simulink model "flightControlSystem"  (R2022b)
settings: Solver=ode3  StartTime=0  StopTime=TFinal  FixedStep=Ts  RelTol=1e-3  EnableMultiTasking=on
undefined symbols (not defined in the file): codertarget, Controller, DiscIntNeverNeededParam, Discrete, Estimator, g, init, Sensors, Time, Ts, var_acc_angle_N, var_bias_gyr_N, var_gyro_p_N, Vehicle
libraries: simulink x38, ctrlSharedLib x4, sharedtransform x3, pid_lib x2, slpidlib x2, parrotlib x1
(part 3 of 3)

== system flightControlSystem/Control System/State Estimator/XY Position Estimator/EstimatorVelocity/AccelerationHandling ==
  dxy_estimin : Inport
  sensorIMU_datin : Inport  Port=2
  orient_estimin : Inport  Port=3
  Z_estimin : Inport  Port=4
  Add : Sum  Inputs=-+
  Bus Selector1 : BusSelector  OutputSignals=ddx,ddy,ddz
  Deactivate Acceleration If OF is not used due to low altitude : simulink/Logic and Bit Operations/Compare To Constant  relop=<=  const=Estimator.pos.opticalFlowZMax  OutDataTypeStr=boolean
  Logical Operator : Logic  Operator=OR  AllPortsSameDT=off  OutDataTypeStr=boolean
  Mux6 : Mux  Inputs=3
  Product : Product  Inputs=3
  Product1 : Product  Multiplication=Matrix(*)
  Rotation Angles to Direction Cosine Matrix : sharedtransform/Rotation Angles to Direction Cosine Matrix  rotationOrder=ZYX  aMode=aMode
  SelectPlanarddxy : Selector  InputPortWidth=3  IndexOptions=Index vector (dialog)  Indices=[1 2]  OutputSizes=1
  Selector : Selector  InputPortWidth=2  IndexOptions=Index vector (dialog)  Indices=1  OutputSizes=1
  Selector1 : Selector  InputPortWidth=2  IndexOptions=Index vector (dialog)  Indices=2  OutputSizes=1
  do not use acc if optical flow never available (Note OF@60Hz but ZOH to 200!) : simulink/Logic and Bit Operations/Compare To Constant  relop=~=  const=0  OutDataTypeStr=boolean
  do not use acc if optical flow never available (Note OF@60Hz but ZOH to 200!)1 : simulink/Logic and Bit Operations/Compare To Constant  relop=~=  const=0  OutDataTypeStr=boolean
  gainaccinput1 : Gain  OutDataTypeStr=single
  gravity : Constant  Value=[0 0 -g]
  acceleration_world : Outport  OutDataTypeStr=single  VectorParamsAs1DForOutWhenUnconnected=off
  wires:
  do not use acc if optical flow never available (Note OF@60Hz but ZOH to 200!)1/1 -> Logical Operator/2
  do not use acc if optical flow never available (Note OF@60Hz but ZOH to 200!)/1 -> Logical Operator/1
  Logical Operator/1 -> Product/1
  Selector1/1 -> do not use acc if optical flow never available (Note OF@60Hz but ZOH to 200!)1/1
  Selector/1 -> do not use acc if optical flow never available (Note OF@60Hz but ZOH to 200!)/1
  dxy_estimin/1 -> Selector1/1, Selector/1
  Product/1 -> acceleration_world/1
  Deactivate Acceleration If OF is not used due to low altitude/1 -> Product/3
  Z_estimin/1 -> Deactivate Acceleration If OF is not used due to low altitude/1
  Add/1 -> SelectPlanarddxy/1
  Product1/1 -> Add/1
  gravity/1 -> Product1/2
  SelectPlanarddxy/1 -> gainaccinput1/1
  Bus Selector1/3 -> Mux6/3  "<ddz>"
  Bus Selector1/1 -> Mux6/1  "<ddx>"
  sensorIMU_datin/1 -> Bus Selector1/1
  Mux6/1 -> Add/2
  Bus Selector1/2 -> Mux6/2  "<ddy>"
  orient_estimin/1 -> Rotation Angles to Direction Cosine Matrix/1
  Rotation Angles to Direction Cosine Matrix/1 -> Product1/1
  gainaccinput1/1 -> Product/2

== system flightControlSystem/Control System/State Estimator/XY Position Estimator/EstimatorVelocity/Angular velocity compensation for optical flow ==
  note: Optical flow readings are affected by both linear and angular velocity of the drone. We need to subtract the effect of angular velocity before using the flow data
  z_estimate : Inport
  Angular velocity w/o bias : Inport  Port=2
  Abs : Abs  SaturateOnIntegerOverflow=off
  Data Type Conversion : DataTypeConversion  SaturateOnIntegerOverflow=off  RndMeth=Floor
  Demux : Demux  Outputs=2
  Gain1 : Gain  Gain=-1
  Mux : Mux  Inputs=2
  Selector : Selector  InputPortWidth=3  IndexOptions=Index vector (dialog)  Indices=[1 2]  OutputSizes=1
  prod : Product  Inputs=**
  angular velocity correction : Outport
  wires:
  Gain1/1 -> Mux/1
  Mux/1 -> Data Type Conversion/1
  Demux/2 -> Gain1/1
  Data Type Conversion/1 -> angular velocity correction/1
  prod/1 -> Demux/1
  z_estimate/1 -> Abs/1
  Demux/1 -> Mux/2
  Selector/1 -> prod/2
  Abs/1 -> prod/1
  Angular velocity w/o bias/1 -> Selector/1

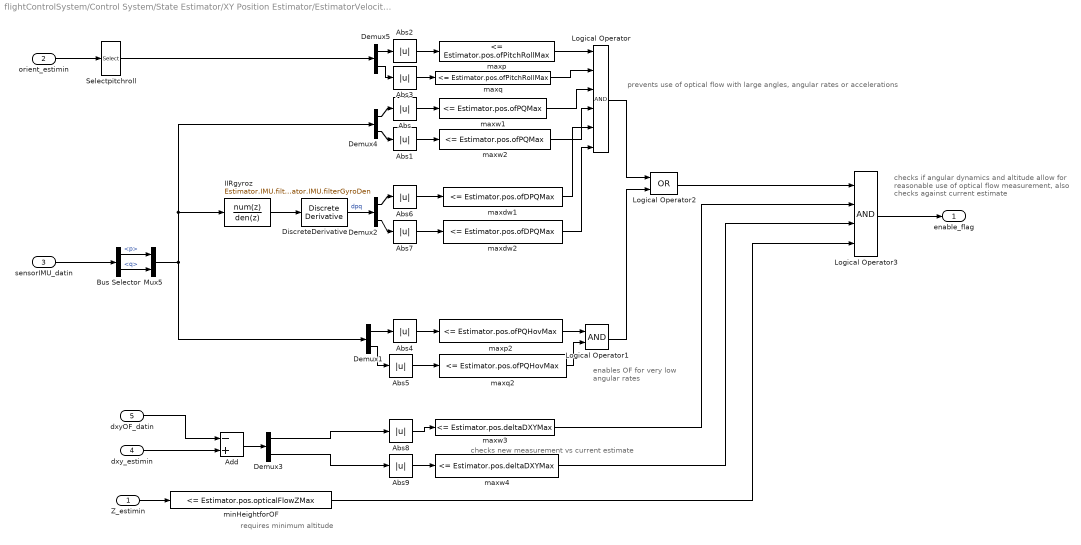
== system flightControlSystem/Control System/State Estimator/XY Position Estimator/EstimatorVelocity/DataHandling ==
  note: prevents use of optical flow with large angles, angular rates or accelerations
  note: enables OF for very
      | low angular rates
  note: checks if angular dynamics and altitude allow for
      | reasonable use of optical flow measurement,
      | also checks against current estimate
  note: checks new measurement vs current estimate
  note: requires minimum altitude
  Z_estimin : Inport
  orient_estimin : Inport  Port=2
  sensorIMU_datin : Inport  Port=3
  dxy_estimin : Inport  Port=4
  dxyOF_datin : Inport  Port=5
  Abs{,1..9} (10 alike) : Abs  SaturateOnIntegerOverflow=off
  Add : Sum  Inputs=-+
  Bus Selector : BusSelector  OutputSignals=p,q
  Demux{1..5} (5 alike) : Demux  Outputs=2
  DiscreteDerivative : simulink/Discrete/Discrete Derivative  gainval=1.0  ICPrevScaledInput=0.0  OutMin=[]  OutMax=[]  OutDataType=fixdt(1, 16)  OutScaling=2^-10  DoSatur=off
  IIRgyroz : DiscreteFilter  Numerator=Estimator.IMU.filterGyroNum  Denominator=Estimator.IMU.filterGyroDen
  Logical Operator : Logic  Inputs=6  AllPortsSameDT=off  OutDataTypeStr=boolean
  Logical Operator1 : Logic  AllPortsSameDT=off  OutDataTypeStr=boolean
  Logical Operator2 : Logic  Operator=OR  AllPortsSameDT=off  OutDataTypeStr=boolean
  Logical Operator3 : Logic  Inputs=4  AllPortsSameDT=off  OutDataTypeStr=boolean
  Mux5 : Mux  Inputs=2
  Selectpitchroll : Selector  InputPortWidth=3  IndexOptions=Index vector (dialog)  Indices=[2 3]  OutputSizes=1
  maxdw1 : simulink/Logic and Bit Operations/Compare To Constant  relop=<=  const=Estimator.pos.ofDPQMax  OutDataTypeStr=boolean
  maxdw2 : simulink/Logic and Bit Operations/Compare To Constant  relop=<=  const=Estimator.pos.ofDPQMax  OutDataTypeStr=boolean
  maxp : simulink/Logic and Bit Operations/Compare To Constant  relop=<=  const=Estimator.pos.ofPitchRollMax  OutDataTypeStr=boolean
  maxp2 : simulink/Logic and Bit Operations/Compare To Constant  relop=<=  const=Estimator.pos.ofPQHovMax  OutDataTypeStr=boolean
  maxq : simulink/Logic and Bit Operations/Compare To Constant  relop=<=  const=Estimator.pos.ofPitchRollMax  OutDataTypeStr=boolean
  maxq2 : simulink/Logic and Bit Operations/Compare To Constant  relop=<=  const=Estimator.pos.ofPQHovMax  OutDataTypeStr=boolean
  maxw1 : simulink/Logic and Bit Operations/Compare To Constant  relop=<=  const=Estimator.pos.ofPQMax  OutDataTypeStr=boolean
  maxw2 : simulink/Logic and Bit Operations/Compare To Constant  relop=<=  const=Estimator.pos.ofPQMax  OutDataTypeStr=boolean
  maxw3 : simulink/Logic and Bit Operations/Compare To Constant  relop=<=  const=Estimator.pos.deltaDXYMax  OutDataTypeStr=boolean
  maxw4 : simulink/Logic and Bit Operations/Compare To Constant  relop=<=  const=Estimator.pos.deltaDXYMax  OutDataTypeStr=boolean
  minHeightforOF : simulink/Logic and Bit Operations/Compare To Constant  relop=<=  const=Estimator.pos.opticalFlowZMax  OutDataTypeStr=boolean
  enable_flag : Outport  VectorParamsAs1DForOutWhenUnconnected=off
  wires:
  minHeightforOF/1 -> Logical Operator3/4
  IIRgyroz/1 -> DiscreteDerivative/1
  Mux5/1 -> Demux1/1, Demux4/1, IIRgyroz/1
  maxw4/1 -> Logical Operator3/3
  maxw3/1 -> Logical Operator3/2
  dxyOF_datin/1 -> Add/1
  Demux3/2 -> Abs9/1
  Demux3/1 -> Abs8/1
  dxy_estimin/1 -> Add/2
  Add/1 -> Demux3/1
  Abs9/1 -> maxw4/1
  Abs8/1 -> maxw3/1
  Logical Operator2/1 -> Logical Operator3/1
  Logical Operator3/1 -> enable_flag/1
  DiscreteDerivative/1 -> Demux2/1  "dpq"
  Demux2/2 -> Abs7/1
  Demux2/1 -> Abs6/1
  Abs7/1 -> maxdw2/1
  Abs6/1 -> maxdw1/1
  Logical Operator1/1 -> Logical Operator2/2
  Demux1/2 -> Abs5/1
  Demux1/1 -> Abs4/1
  Abs5/1 -> maxq2/1
  Abs4/1 -> maxp2/1
  Abs3/1 -> maxq/1
  Abs2/1 -> maxp/1
  Demux4/2 -> Abs1/1
  Demux4/1 -> Abs/1
  Abs1/1 -> maxw2/1
  Abs/1 -> maxw1/1
  Z_estimin/1 -> minHeightforOF/1
  Logical Operator/1 -> Logical Operator2/1
  maxw1/1 -> Logical Operator/3
  Bus Selector/1 -> Mux5/1  "<p>"
  Selectpitchroll/1 -> Demux5/1
  sensorIMU_datin/1 -> Bus Selector/1
  maxq2/1 -> Logical Operator1/2
  Bus Selector/2 -> Mux5/2  "<q>"
  maxp/1 -> Logical Operator/1
  maxw2/1 -> Logical Operator/4
  orient_estimin/1 -> Selectpitchroll/1
  maxdw1/1 -> Logical Operator/5
  maxdw2/1 -> Logical Operator/6
  maxq/1 -> Logical Operator/2
  Demux5/1 -> Abs2/1
  Demux5/2 -> Abs3/1
  maxp2/1 -> Logical Operator1/1

== system flightControlSystem/Control System/State Estimator/XY Position Estimator/EstimatorVelocity/xy velocity w//o angular velocity compensation ==
  note: Optical flow raw readings are converted to velocity in m/s based on the estimated altitude
  optical_flow : Inport
  z_estimate : Inport  Port=2
  " " : Product  Inputs=**
  Compare To Constant : simulink/Logic and Bit Operations/Compare To Constant  relop=<  const=200*4  OutDataTypeStr=boolean
  Counter Free-Running : simulink/Sources/Counter Free-Running  NumBits=32  tsamp=-1
  Gain : Gain  Gain=-1
  Select dxy : Selector  InputPortWidth=3  IndexOptions=Index vector (dialog)  Indices=[1 2]  OutputSizes=1
  Switch : Switch  Criteria=u2 > Threshold  SaturateOnIntegerOverflow=off  InputSameDT=off
  opticalFlowErrorCorrect : Gain  Gain=1.15
  optical_flow_dx_dy : Outport
  wires:
  Select dxy/1 -> optical_flow_dx_dy/1  "optical_flow_dx_dy"
  " "/1 -> opticalFlowErrorCorrect/1
  opticalFlowErrorCorrect/1 -> Switch/3
  Gain/1 -> " "/2
  Switch/1 -> Select dxy/1
  Counter Free-Running/1 -> Compare To Constant/1
  Compare To Constant/1 -> Switch/2
  optical_flow/1 -> " "/1, Switch/1
  z_estimate/1 -> Gain/1

== matlab function flightControlSystem/Control System/my_old_version/MATLAB Function ==
  data: mode input; new_mode output; temp input; temp_out output; angle input
function [new_mode, temp_out] = fcn(mode, temp, angle)
temp_out = temp;

if mode == 2
    temp_out = max(mode, temp_out);
    
elseif temp_out == 2 && mode ~= 2
    temp_out = 2;
    
elseif mode == 1 && abs(angle) < 10
    temp_out = 0;
    
else
    temp_out = mode;
end

new_mode = temp_out;

== matlab function flightControlSystem/Control System/my_old_version/MATLAB Function1 ==
  data: x_1 input; x_coord output; y_1 input; mode input; x_2 input; y_2 input; y_coord output; x_3 input; y_3 input; z_3 input; z_coord output
function [x_coord, y_coord, z_coord] = fcn(x_1, y_1, mode, x_2, y_2, x_3, y_3, z_3)

if mode == 0
    x_coord = x_1;
    y_coord = y_1;
    z_coord = -1.1;
    
elseif mode == 1
    x_coord = x_2;
    y_coord = y_2;
    z_coord = -1.1;

% elseif mode == 1 && y_2 >= y_1
%     x_coord = x_2;
%     y_coord = y_2;
%     z_coord = -1.1;
%     
% elseif mode == 1 && y_1 < 0 && y_2 < 0 && y_1 <= y_2
%     x_coord = x_2;
%     y_coord = y_1;
%     z_coord = -1.1;
%     
% elseif mode == 1 && y_1 < 0 && y_2 < 0 && y_2 <= y_1
%     x_coord = x_2;
%     y_coord = y_2;
%     z_coord = -1.1;
%     
% elseif mode == 1 && y_1 > 0 && y_2 < 0
%     disp("condiiton1:");
%     x_coord = x_2;
%     y_coord = y_2;
%     z_coord = -1.1;
%     
% elseif mode == 1 && y_1 < 0 && y_2 > 0
%     disp("consition2:");
%     x_coord = x_2;
%     y_coord = y_2;
%     z_coord = -1.1;
%     
elseif mode == 2
    x_coord = x_3;
    y_coord = y_3;
    z_coord = z_3;
    
else
    x_coord = x_2;
    y_coord = y_2;
    z_coord = z_3;
end

== matlab function flightControlSystem/Control System/my_old_version/MATLAB Function2 ==
  data: angle input; final output; mode input; read_in input
function final = fcn(angle, mode, read_in)

if mode == 2
    final = 2;
    
elseif abs(angle) >= 90 || read_in ~= 0
    final = 1;
   
else
    final = mode;
end

== matlab function flightControlSystem/Control System/my_old_version/MATLAB Function3 ==
  data: mode input; bool_in input; y_out output
function y_out = fcn(mode, bool_in)

if mode == 2
    y_out = 2;
elseif bool_in == 1
    y_out = 1;
elseif bool_in == 0
    y_out = 0;
else
    y_out = 2;
end

== matlab function flightControlSystem/Control System/my_old_version/Switch Case II/MATLAB Function ==
  data: angle input; x_coord output; move_x input; move_y input; x_signal input; y_signal input; y_coord output; x_move output; y_move output; count_in input; count_out output; temp_in input; temp_out output; max_angle_in input; max_angle_out output
function [x_coord, y_coord, x_move, y_move, count_out, temp_out, max_angle_out] = fcn(angle, move_x, move_y, x_signal, y_signal, count_in, temp_in, max_angle_in)
temp_out = temp_in;
% max_angle_out = max_angle_in;
% max_angle_out = max(abs(angle), max_angle_out);
% temp_out = 450;
% disp(max_angle_in);
% disp(angle);

if count_in == 0
    temp_out = 400;
    max_angle_out = angle;
    x_coord = x_signal;
    y_coord = y_signal;
    x_move = move_x;
    y_move = move_y;
    count_out = count_in + 1;    

elseif ((count_in < temp_out) || (count_in > temp_out && count_in < 3*temp_out)) 
    x_coord = x_signal + move_x;
    y_coord = y_signal + move_y;
    x_move = move_x;
    y_move = move_y;
    count_out = count_in + 1;
    max_angle_out = max_angle_in;
    
elseif count_in == temp_out
    x_move = cos(max_angle_in*pi/180)*0.0005;
    y_move = sin(max_angle_in*pi/180)*0.0005;
    count_out = temp_out+1;
    x_coord = x_signal;
    y_coord = y_signal;
    max_angle_out = max_angle_in;
    
else
   x_coord = x_signal;
   y_coord = y_signal;
   x_move = move_x;
   y_move = move_y;
   count_out = 0;
   max_angle_out = max_angle_in;
end

== matlab function flightControlSystem/Control System/my_old_version/Switch Case III/MATLAB Function ==
  data: x_signal input; x_coord output; y_signal input; z_signal input; move_x input; move_y input; temp_in input; y_coord output; z_coord output; temp_out output
function [x_coord, y_coord, z_coord, temp_out] = fcn(x_signal, y_signal, z_signal, move_x, move_y, temp_in)

if temp_in < 445
    x_coord = x_signal + move_x;
    y_coord = y_signal + move_y;
    z_coord = z_signal;
    temp_out = temp_in + 1;
 
else
    x_coord = x_signal;
    y_coord = y_signal;
    z_coord = z_signal + 0.0005;
    temp_out = temp_in;
end

== matlab function flightControlSystem/Control System/Path Planning/MATLAB Function3 ==
  data: mode input; bool_in input; y_out output
function y_out = fcn(mode, bool_in)

if mode == 2
    y_out = 2;
elseif bool_in == 1
    y_out = 1;
elseif bool_in == 0
    y_out = 0;
else
    y_out = 2;
end

== matlab function flightControlSystem/Control System/Controller/Position Controller/Position error transformation (Earth to Body frame) ==
  data: yaw input; xy_err_earth input; xy_err_body output
function xy_err_body = fcn(yaw,xy_err_earth)

transformation = [cos(yaw), sin(yaw); -sin(yaw),  cos(yaw)];
xy_err_body = transformation * xy_err_earth;


end

== matlab function flightControlSystem/Image Processing System/Image Processing Function ==
  data: image input; output_angle output; mode output
%%
% The hough transform generates the angle and bins. We use the bin angles
% to determine the flow of gradients. Use that angle to perform path
% planning. 

% Steps : 
% 1. Use canny edge detector to detemine edges of the path as well as the
% circle. 
% 2. Use hough transform, followed by houghlines to determine the peaks and
% four parameters i.e. points1, points2, theta, rho. 
% 3. Use houghlines to draw the lines. 
% 3. Use the theta to compare angles. 

%% Implementation

function [output_angle, mode] = fcn(image)


angle = 0;
mode = 0;
angle_temp = 0;
temp = false;
temp_ = 0;

% Binarize and edge detection 
binary_img = imbinarize(image);
canny_output = edge(binary_img,'canny');
morphed_output = bwmorph(canny_output,'thin',Inf);

% find circles finds circular edges 
centers = imfindcircles(binary_img,[15 40]);

% Hough transform for detecting lane lines 
[H,T,R] = hough(morphed_output,'Theta',-90:1:89);
P = houghpeaks(H,5,'threshold',ceil(0.3*max(H(:))));
lines = houghlines(canny_output,T,R,P,'FillGap',5,'MinLength',10);


max_angle = 0;
min_angle = 0;
for i = 1:length(lines)
    max_angle = max([max_angle,lines(i).theta]);
    min_angle = min([min_angle, lines(i).theta]);
end

if length(lines) == 4  % 화면에 Red Line이 포착된다면 조건문 만족
    mode = 1;
    for i = 1:length(lines)
        hough_angle = lines(i).theta;
        if (hough_angle > angle_temp - 10) || (hough_angle < angle_temp + 10)
            angle = lines(i).theta;    
            temp_ = sign(lines(i).point1(1) + angle);
        end
        if temp == false
            temp = true;
            angle_temp = angle;
        end
    end
    
    if angle < 0 && temp_ == 1
        angle = angle + 180;
    elseif angle > 0 && temp_ == -1
        angle = angle - 180;
    end
end

if length(centers) == 2
    mode = 2;
end

output_angle = angle;

== matlab function flightControlSystem/Control System/Path Planning/MATLAB Function1 ==
  data: x_1 input; x_coord output; y_1 input; mode input; x_2 input; y_2 input; y_coord output; x_3 input; y_3 input; z_3 input; z_coord output
function [x_coord, y_coord, z_coord] = fcn(x_1, y_1, mode, x_2, y_2, x_3, y_3, z_3)

if mode == 0
    x_coord = x_1;
    y_coord = y_1;
    z_coord = -1.1;
    
elseif mode == 1
    x_coord = x_2;
    y_coord = y_2;
    z_coord = -1.1;

% elseif mode == 1 && y_2 >= y_1
%     x_coord = x_2;
%     y_coord = y_2;
%     z_coord = -1.1;
%     
% elseif mode == 1 && y_1 < 0 && y_2 < 0 && y_1 <= y_2
%     x_coord = x_2;
%     y_coord = y_1;
%     z_coord = -1.1;
%     
% elseif mode == 1 && y_1 < 0 && y_2 < 0 && y_2 <= y_1
%     x_coord = x_2;
%     y_coord = y_2;
%     z_coord = -1.1;
%     
% elseif mode == 1 && y_1 > 0 && y_2 < 0
%     disp("condiiton1:");
%     x_coord = x_2;
%     y_coord = y_2;
%     z_coord = -1.1;
%     
% elseif mode == 1 && y_1 < 0 && y_2 > 0
%     disp("consition2:");
%     x_coord = x_2;
%     y_coord = y_2;
%     z_coord = -1.1;
%     
elseif mode == 2
    x_coord = x_3;
    y_coord = y_3;
    z_coord = z_3;
    
else
    x_coord = x_2;
    y_coord = y_2;
    z_coord = z_3;
end

== matlab function flightControlSystem/Control System/Path Planning/MATLAB Function ==
  data: mode input; new_mode output; temp input; temp_out output; angle input
function [new_mode, temp_out] = fcn(mode, temp, angle)
temp_out = temp;

if mode == 2
    temp_out = max(mode, temp_out);
    
elseif temp_out == 2 && mode ~= 2
    temp_out = 2;
    
elseif mode == 1 && abs(angle) < 10
    temp_out = 0;
    
else
    temp_out = mode;
end

new_mode = temp_out;

== matlab function flightControlSystem/Control System/Path Planning/Switch Case II/MATLAB Function ==
  data: angle input; x_coord output; move_x input; move_y input; x_signal input; y_signal input; y_coord output; x_move output; y_move output; count_in input; count_out output; temp_in input; temp_out output; max_angle_in input; max_angle_out output
function [x_coord, y_coord, x_move, y_move, count_out, temp_out, max_angle_out] = fcn(angle, move_x, move_y, x_signal, y_signal, count_in, temp_in, max_angle_in)
temp_out = temp_in;
% max_angle_out = max_angle_in;
% max_angle_out = max(abs(angle), max_angle_out);
% sign_ = sign(angle);

% temp_out = 450;
% disp(max_angle_in);
% disp(angle);
if count_in == 0
    
    temp_out = (450/90)*abs(angle - max_angle_in);
    max_angle_out = angle;
    x_coord = x_signal;
    y_coord = y_signal;
    x_move = move_x;
    y_move = move_y;
    count_out = count_in + 1;    

elseif ((count_in < temp_out) || (count_in > temp_out && count_in < 3*temp_out)) 
    x_coord = x_signal + move_x;
    y_coord = y_signal + move_y;
    x_move = move_x;
    y_move = move_y;
    count_out = count_in + 1;
    max_angle_out = max_angle_in;
    
elseif count_in == temp_out
    x_move = cos(max_angle_in*pi/180)*0.0005;
    y_move = sin(max_angle_in*pi/180)*0.0005;
    count_out = temp_out+1;
    x_coord = x_signal;
    y_coord = y_signal;
    max_angle_out = max_angle_in;
    
else
   x_coord = x_signal;
   y_coord = y_signal;
   x_move = move_x;
   y_move = move_y;
   count_out = 0;
   max_angle_out = max_angle_in;
end

== matlab function flightControlSystem/Control System/Path Planning/Switch Case III/MATLAB Function ==
  data: x_signal input; x_coord output; y_signal input; z_signal input; move_x input; move_y input; temp_in input; y_coord output; z_coord output; temp_out output
function [x_coord, y_coord, z_coord, temp_out] = fcn(x_signal, y_signal, z_signal, move_x, move_y, temp_in)

if temp_in < 500
    x_coord = x_signal + move_x;
    y_coord = y_signal + move_y;
    z_coord = z_signal;
    temp_out = temp_in + 1;
 
else
    x_coord = x_signal;
    y_coord = y_signal;
    z_coord = z_signal + 0.0005;
    temp_out = temp_in;
end

== matlab function flightControlSystem/Control System/Path Planning/MATLAB Function2 ==
  data: angle input; final output; mode input; read_in input
function final = fcn(angle, mode, read_in)

if mode == 2
    final = 2;
    
elseif abs(angle) >= 90 || read_in ~= 0
    final = 1;
   
else
    final = mode;
end
